simulink model "e9_16"  (R2016a)
settings: Solver=VariableStepAuto  SolverMode=SingleTasking  StartTime=0.0  StopTime=.2  RelTol=1e-3
libraries: spsIGBTDiodeLib x4, spsVoltageMeasurementLib x2, spsACVoltageSourceLib x1, spsCurrentMeasurementLib x1, spsDCVoltageSourceLib x1, spsPLLLib x1, spsSeriesRLCBranchLib x1, spspowerguiLib x1
settings Model: Creator=Asus  LastModifiedBy=Asus
settings DataIOCC: ReturnWorkspaceOutputs=on
settings DebuggingCC: SFUnexpectedBacktrackingDiag=error  SFNoUnconditionalDefaultTransitionDiag=error
settings SFSimCC: SimUseLocalCustomCode=on
settings RTWCC: RTWUseLocalCustomCode=on
settings GRTTargetCC: TargetLangStandard=C99 (ISO)
settings ConfigComp: CovMetricSettings=dwe  CovSaveCumulativeToWorkspaceVar=off  CovSaveSingleToWorkspaceVar=off  CovExternalEMLEnable=on

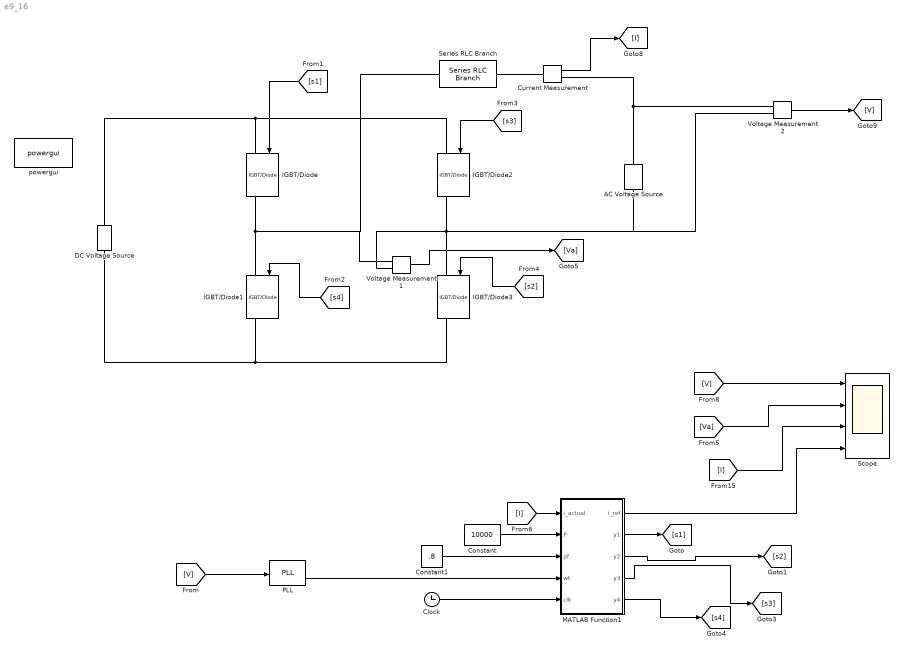
== system e9_16 ==
  AC Voltage Source : spsACVoltageSourceLib/AC Voltage Source  Amplitude=220  Phase=0  Frequency=50  SampleTime=0  Measurements=None  BusType=swing  Pref=10e3  Qref=0  Qmin=-inf  Qmax=+inf
  Clock : Clock
  Constant : Constant  Value=10000
  Constant1 : Constant  Value=.8
  Current Measurement : spsCurrentMeasurementLib/Current Measurement  PhasorSimulation=off  OutputType=Complex  PSBequivalent=0
  DC Voltage Source : spsDCVoltageSourceLib/DC Voltage Source  Amplitude=400  Measurements=None
  IGBT/Diode{,1..3} (4 alike) : spsIGBTDiodeLib/IGBT//Diode  Ron=1e-3  Rs=1e5  Cs=inf  Measurements=on
  MATLAB Function1 : MATLAB Function  TreatAsAtomicUnit=on
  PLL : spsPLLLib/PLL  Fmin=50  Par_Init=[0, 50]  ParK=[180, 3200, 1]  TcD=1e-4  MaxRateChangeFreq=12  FilterCutOffFreq=25  Ts=0  AGC=on
  Scope : Scope  NumInputPorts=4
  Series RLC Branch : spsSeriesRLCBranchLib/Series RLC Branch  LConnTagsString=__new0  RConnTagsString=__new0  BranchType=RL  Resistance=.1  Inductance=10e-3  SetiL0=off  InitialCurrent=0  Capacitance=1e-6  Setx0=off  InitialVoltage=0  Measurements=None
  Voltage Measurement1 : spsVoltageMeasurementLib/Voltage Measurement  PhasorSimulation=off  OutputType=Complex  PSBequivalent=0
  Voltage Measurement2 : spsVoltageMeasurementLib/Voltage Measurement  PhasorSimulation=off  OutputType=Complex  PSBequivalent=0
  powergui : spspowerguiLib/powergui  Priority=1  SimulationMode=Discrete  SampleTime=50e-6  frequency=60  Iterations=50  frequencyindice=0  Pbase=100e6  ErrMax=1e-4  UnitsV=kV  UnitsW=MW  buscounter=0  FunctionMessages=off  echomessages=off  EnableUseOfTLC=off  CurrentSourceSwitches=off  DisableSnubberDevices=off  DisableRonSwitches=off  DisableVfSwitches=off  DisplayEquations=off  AutomaticDiscreteSolvers=off  SolverType=Tustin/Backward Euler (TBE)  Interpol=off  ExternalGateDelay=off  methode=off  Ts=100  x0status=blocks  SPID=on  SwTol=0  HookPort=off  NonlinearTolerance=1e-4  nMaxIteration=100  ContinueOnMaxIteration=off  RestoreLinks=warning  ResistiveCurrentMeasurement=off  Frange=[0:2:500]  Ylog=off  Xlog=on  ShowGrid=off  save=off  variable=ZData  structure=0  ZoomFFT=off  StartTime=0.0  cycles=1  DisplayStyle=1  fundamental=60  FreqAxis=off  MaxFrequency=1000  frequencyindicesteady=1  RmsSteady=1  display=off
  wires:
  Voltage Measurement2/1 -> [V]
  [s2] -> IGBT/Diode3/1
  [s3] -> IGBT/Diode2/1
  [s1] -> IGBT/Diode/1
  [s4] -> IGBT/Diode1/1
  [V] -> Scope/1
  Current Measurement/1 -> [I]
  [I] -> MATLAB Function1/1(i_actual)
  MATLAB Function1/2(y1) -> [s1]
  MATLAB Function1/3(y2) -> [s2]
  MATLAB Function1/4(y3) -> [s3]
  MATLAB Function1/5(y4) -> [s4]
  Constant/1 -> MATLAB Function1/2(P)
  Constant1/1 -> MATLAB Function1/3(pf)
  [V] -> PLL/1
  PLL/2 -> MATLAB Function1/4(wt)
  Clock/1 -> MATLAB Function1/5(clk)
  MATLAB Function1/1(i_ref) -> Scope/4
  [Va] -> Scope/2
  [I] -> Scope/3
  Voltage Measurement1/1 -> [Va]
  connections:
  IGBT/Diode3/RConn1 -- DC Voltage Source/LConn1 -- IGBT/Diode1/RConn1
  DC Voltage Source/RConn1 -- IGBT/Diode/LConn1 -- IGBT/Diode2/LConn1
  IGBT/Diode2/RConn1 -- Voltage Measurement2/LConn2 -- AC Voltage Source/LConn1 -- Voltage Measurement1/LConn2 -- IGBT/Diode3/LConn1
  IGBT/Diode/RConn1 -- Voltage Measurement1/LConn1 -- Series RLC Branch/RConn1 -- IGBT/Diode1/LConn1
  Current Measurement/LConn1 -- Series RLC Branch/LConn1
  Current Measurement/RConn1 -- AC Voltage Source/RConn1 -- Voltage Measurement2/LConn1

== matlab function e9_16/MATLAB Function1 ==
  settings: updateMethod=DISCRETE
  data: i_actual input; i_ref output; P input; pf input; wt input; clk input; y1 output; y2 output; y3 output; y4 output
function [i_ref,y1,y2,y3,y4] = fcn(i_actual,P,pf,wt,clk) 
P1=P;
Vg=220;
P2=P/2;
A=acos(pf); 

if clk<0.1 
    ig_m=(P1*sqrt(2))/(Vg*pf); 
    ig=ig_m*sin(wt-A); 
    i_ref = ig; 
else 
    ig_m=(P2*sqrt(2))/(Vg*pf); 
    ig=ig_m*sin(wt-A); 
    i_ref = ig; 
end 
persistent s1 
if isempty(s1) 
    s1=0; 
end 
persistent s2 
if isempty(s2) 
    s2=0; 
end 
persistent s3 
if isempty(s3) 
    s3=0; 
end 
persistent s4 
if isempty(s4) 
    s4=0; 
end 
d=1; 
e=i_actual-i_ref; 
if i_ref>=0 
    if e<-d 
        s1=1; s2=1; s3=0; s4=0; 
    elseif e>d 
        s1=0; s2=0; s3=1; s4=1; 
    end 
else 
    if e<-d 
        s1=1; s2=1; s3=0; s4=0; 
    elseif e>d 
        s1=0; s2=0; s3=1; s4=1; 
    end 
end 
y1=s1; 
y2=s2; 
y3=s3; 
y4=s4; 
end
